simulink model "BlockDiagram_DCmotor_lecture20_control1"  (R2019a)
settings: Solver=VariableStepAuto  StartTime=0.0  StopTime=1  RelTol=1e-3
values from neighbouring files (symbols this model uses):
  Jeq = 1    [DCmotor_InputData.m]    (also in DCmotor_InputData_lecture20.m = 0.0022; DCmotor_InputData_lecture20_control1.m = 0.0022; DCmotor_InputData_lecture20_control_study.m = 0.0022; DCmotor_InputData_lecture20_loadLin.m = 0.0022)
  kE = 0.5    [DCmotor_InputData.m]    (also in DCmotor_InputData_lecture20.m = 0.129; DCmotor_InputData_lecture20_control1.m = 0.129; DCmotor_InputData_lecture20_control_study.m = 0.129; DCmotor_InputData_lecture20_loadLin.m = 0.129)
  kI = kP * sm    [DCmotor_InputData_lecture20_control1.m]    (also in DCmotor_InputData_lecture20_control_study.m)
  kP = 200    [DCmotor_InputData_lecture20_control1.m]    (also in DCmotor_InputData_lecture20_control_study.m)
  kT = 0.5    [DCmotor_InputData.m]    (also in DCmotor_InputData_lecture20.m = 0.129; DCmotor_InputData_lecture20_control1.m = 0.129; DCmotor_InputData_lecture20_control_study.m = 0.129; DCmotor_InputData_lecture20_loadLin.m = 0.129)
  La = 0.2    [DCmotor_InputData.m]    (also in DCmotor_InputData_lecture20.m = 0.0072; DCmotor_InputData_lecture20_control1.m = 0.0072; DCmotor_InputData_lecture20_control_study.m = 0.0072; DCmotor_InputData_lecture20_loadLin.m = 0.0072)
  Ra_20 = Ra    (= 0.5)    [DCmotor_InputData_lecture20.m]    (also in DCmotor_InputData_lecture20_control1.m; DCmotor_InputData_lecture20_control_study.m; DCmotor_InputData_lecture20_loadLin.m; DCmotor_InputData_lecture20_loadQuad.m)
  T_Load = 0.5    [DCmotor_InputData_lecture20.m]    (also in DCmotor_InputData_lecture20_control1.m = 0.2)
  Vdc = 24    [DCmotor_InputData_lecture20.m]    (also in DCmotor_InputData_lecture20_control1.m; DCmotor_InputData_lecture20_loadLin.m; DCmotor_InputData_lecture20_loadQuad.m)
  wm_ref = Wm_ref * pi / 30    (= 104.71975512)    [DCmotor_InputData_lecture20_control1.m]
settings Model: Creator=Luca Papini  LastModifiedBy=Luca Papini
settings DataIOCC: SaveFormat=StructureWithTime  SaveState=on

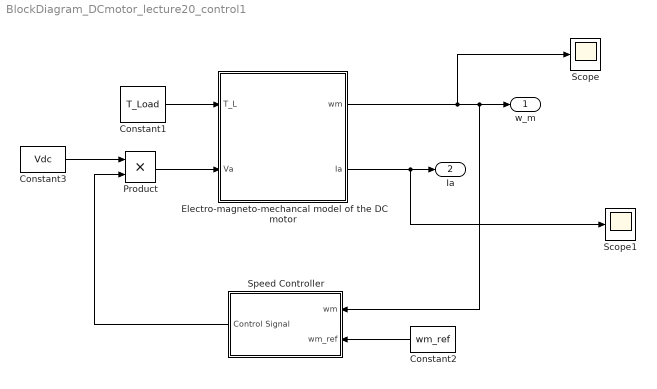
== system BlockDiagram_DCmotor_lecture20_control1 ==
  Constant1 : Constant  Value=T_Load
  Constant2 : Constant  Value=wm_ref
  Constant3 : Constant  Value=Vdc
  Electro-magneto-mechancal model of the DC motor : Subsystem
  Product : Product
  Scope : Scope
  Scope1 : Scope
  Speed Controller : Subsystem
  w_m : Outport
  Ia : Outport  Port=2
  wires:
  Constant1/1 -> Electro-magneto-mechancal model of the DC motor/1(T_L)
  Product/1 -> Electro-magneto-mechancal model of the DC motor/2(Va)
  Speed Controller/1(Control Signal) -> Product/2
  Constant3/1 -> Product/1
  Constant2/1 -> Speed Controller/2(wm_ref)
  Electro-magneto-mechancal model of the DC motor/1(wm) -> Scope/1, Speed Controller/1(wm), w_m/1
  Electro-magneto-mechancal model of the DC motor/2(Ia) -> Scope1/1, Ia/1

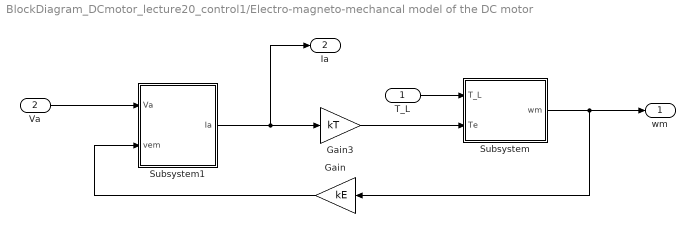
== system BlockDiagram_DCmotor_lecture20_control1/Electro-magneto-mechancal model of the DC motor ==
  T_L : Inport
  Va : Inport  Port=2
  Gain : Gain  Gain=kE
  Gain3 : Gain  Gain=kT
  Subsystem : Subsystem
  Subsystem1 : Subsystem
  wm : Outport
  Ia : Outport  Port=2
  wires:
  Va/1 -> Subsystem1/1(Va)
  Gain3/1 -> Subsystem/2(Te)
  Subsystem/1(wm) -> Gain/1, wm/1
  Gain/1 -> Subsystem1/2(vem)
  Subsystem1/1(Ia) -> Ia/1, Gain3/1
  T_L/1 -> Subsystem/1(T_L)

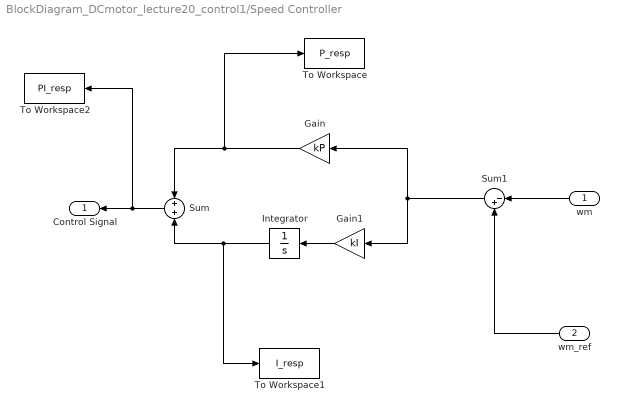
== system BlockDiagram_DCmotor_lecture20_control1/Speed Controller ==
  wm : Inport
  wm_ref : Inport  Port=2
  Gain : Gain  Gain=kP
  Gain1 : Gain  Gain=kI
  Integrator : Integrator  UpperSaturationLimit=1  LowerSaturationLimit=-1
  Sum : Sum  Inputs=+|+
  Sum1 : Sum  Inputs=|-+
  To Workspace : ToWorkspace  VariableName=P_resp  SaveFormat=Structure With Time  SampleTime=-1
  To Workspace1 : ToWorkspace  VariableName=I_resp  SaveFormat=Structure With Time  SampleTime=-1
  To Workspace2 : ToWorkspace  VariableName=PI_resp  SaveFormat=Structure With Time  SampleTime=-1
  Control Signal : Outport
  wires:
  Integrator/1 -> To Workspace1/1, Sum/2
  Gain/1 -> To Workspace/1, Sum/1
  Sum1/1 -> Gain/1, Gain1/1
  Gain1/1 -> Integrator/1
  Sum/1 -> To Workspace2/1, Control Signal/1
  wm/1 -> Sum1/1
  wm_ref/1 -> Sum1/2

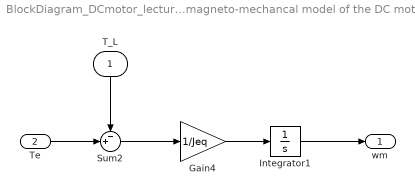
== system BlockDiagram_DCmotor_lecture20_control1/Electro-magneto-mechancal model of the DC motor/Subsystem ==
  T_L : Inport
  Te : Inport  Port=2
  Gain4 : Gain  Gain=1/Jeq
  Integrator1 : Integrator
  Sum2 : Sum  Inputs=-+|
  wm : Outport
  wires:
  Sum2/1 -> Gain4/1
  Integrator1/1 -> wm/1
  T_L/1 -> Sum2/1
  Gain4/1 -> Integrator1/1
  Te/1 -> Sum2/2

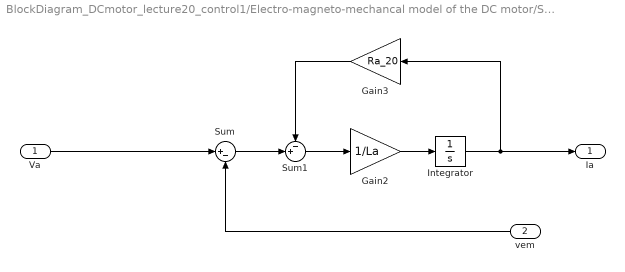
== system BlockDiagram_DCmotor_lecture20_control1/Electro-magneto-mechancal model of the DC motor/Subsystem1 ==
  Va : Inport
  vem : Inport  Port=2
  Gain2 : Gain  Gain=1/La
  Gain3 : Gain  Gain=Ra_20
  Integrator : Integrator
  Sum : Sum  Inputs=|+-
  Sum1 : Sum  Inputs=-+|
  Ia : Outport
  wires:
  Integrator/1 -> Gain3/1, Ia/1
  Gain2/1 -> Integrator/1
  Va/1 -> Sum/1
  Sum1/1 -> Gain2/1
  vem/1 -> Sum/2
  Sum/1 -> Sum1/2
  Gain3/1 -> Sum1/1
